simulink model "test1"  (R2022a)
settings: Solver=FixedStepDiscrete  StartTime=0.0  StopTime=inf  FixedStep=0.01  RelTol=1e-3
libraries: simulink x1
settings Model: Creator=XLI314  LastModifiedBy=XLI314
settings OptimizationCC: DefaultParameterBehavior=Inlined  EnhancedBackFolding=on  PassReuseOutputArgsAs=Individual arguments  ZeroExternalMemoryAtStartup=off  ZeroInternalMemoryAtStartup=off  OptimizeBlockOrder=speed  DifferentSizesBufferReuse=on  OptimizationCustomize=off  EfficientTunableParamExpr=on
settings DebuggingCC: ParameterTunabilityLossMsg=error
settings SFSimCC: MATLABDynamicMemAlloc=off
settings RTWCC: SystemTargetFile=ert.tlc  GenCodeOnly=on  TemplateMakefile=ert_default_tmf  GenerateReport=on  LaunchReport=on
settings CodeAppCC: ForceParamTrailComments=on  IgnoreCustomStorageClasses=off  OperatorAnnotations=on  SimulinkDataObjDesc=on  SFDataObjDesc=on  InsertBlockDesc=on
settings ERTTargetCC: TargetLangStandard=C99 (ISO)  GenerateSampleERTMain=on  InlinedParameterPlacement=NonHierarchical  ERTCustomFileTemplate=example_file_process.tlc

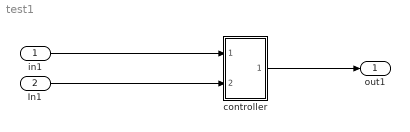
== system test1 ==
  in1 : Inport
  In1 : Inport  Port=2
  controller : Subsystem
  out1 : Outport
  wires:
  in1/1 -> controller/1(In1)
  controller/1(Out1) -> out1/1
  In1/1 -> controller/2(In2)

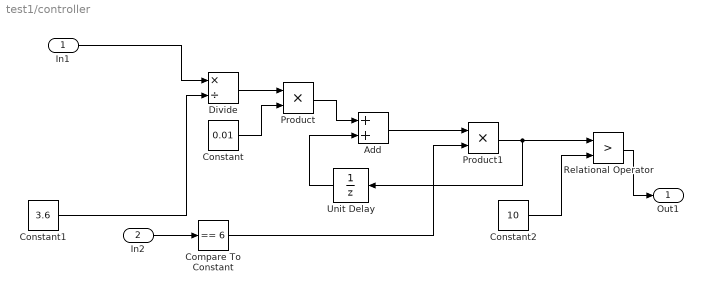
== system test1/controller ==
  In1 : Inport
  In2 : Inport  Port=2
  Add : Sum
  Compare To Constant : simulink/Logic and Bit Operations/Compare To Constant  relop===  const=6  OutDataTypeStr=boolean
  Constant : Constant  Value=0.01
  Constant1 : Constant  Value=3.6
  Constant2 : Constant  Value=10
  Divide : Product  Inputs=*/
  Product : Product
  Product1 : Product
  Relational Operator : RelationalOperator  Operator=>  OutDataTypeStr=boolean  RndMeth=Simplest  InputSameDT=off
  Unit Delay : UnitDelay  SampleTime=-1  HasFrameUpgradeWarning=on
  Out1 : Outport
  wires:
  In2/1 -> Compare To Constant/1
  Constant1/1 -> Divide/2
  In1/1 -> Divide/1
  Constant/1 -> Product/2
  Divide/1 -> Product/1
  Product/1 -> Add/1
  Add/1 -> Product1/1
  Compare To Constant/1 -> Product1/2
  Product1/1 -> Relational Operator/1, Unit Delay/1
  Unit Delay/1 -> Add/2
  Constant2/1 -> Relational Operator/2
  Relational Operator/1 -> Out1/1
